simulink model "pnsequencegeneartor"  (R2021a)
settings: Solver=VariableStepAuto  StartTime=0.0  StopTime=10.0  RelTol=1e-3
settings Model: Creator=GUNA  LastModifiedBy=GUNA

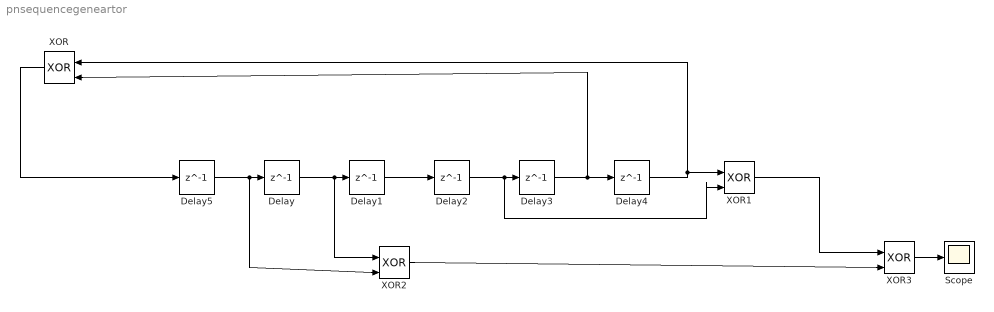
== system pnsequencegeneartor ==
  Delay{,1..5} (6 alike) : Delay  DelayLength=1  InitialCondition=1
  Scope : Scope
  XOR{,1..3} (4 alike) : Logic  Operator=XOR  IconShape=distinctive  AllPortsSameDT=off  OutDataTypeStr=boolean
  wires:
  XOR/1 -> Delay5/1
  Delay5/1 -> XOR2/2, Delay/1
  Delay/1 -> XOR2/1, Delay1/1
  Delay1/1 -> Delay2/1
  Delay2/1 -> XOR1/2, Delay3/1
  Delay3/1 -> XOR/2, Delay4/1
  Delay4/1 -> XOR/1, XOR1/1
  XOR2/1 -> XOR3/2
  XOR1/1 -> XOR3/1
  XOR3/1 -> Scope/1
